simulink model "speedgoat_tcp_io"  (R2023a)
settings: Solver=FixedStepAuto  StartTime=0.0  StopTime=inf  RelTol=1e-3
model workspace (MAT data in the model file):
  outputs = {'uint8', 'uint8', 'uint8', 'uint8', 'uint8', 'uint8', 'uint8', 'uint8', 'double', 'double', 'double', 'double'}
undefined symbols (not defined in the file): Ended, Single
libraries: speedgoatlib_IO191 x5, slrealtimeiplib x3, slrealtimeutilitieslib x1, etargetslib x1
settings Model: Creator=tyler  LastModifiedBy=ivanl
settings SolverCC: ConcurrentTasks=on  PositivePriorityOrder=on
settings OptimizationCC: BlockReduction=off  OptimizeBlockIOStorage=off
settings DebuggingCC: TasksWithSamePriorityMsg=none
settings HardwareCC: ProdBitPerLong=64  ProdLongLongMode=on  ProdHWDeviceType=Intel->x86-64 (Linux 64)
settings RTWCC: Description=Simulink Real-Time  SystemTargetFile=slrealtime.tlc  TemplateMakefile=slrealtime_default_tmf  Toolchain=Simulink Real-Time Toolchain  BuildConfiguration=Faster Runs  CodeExecutionProfiling=on  TargetLang=C++

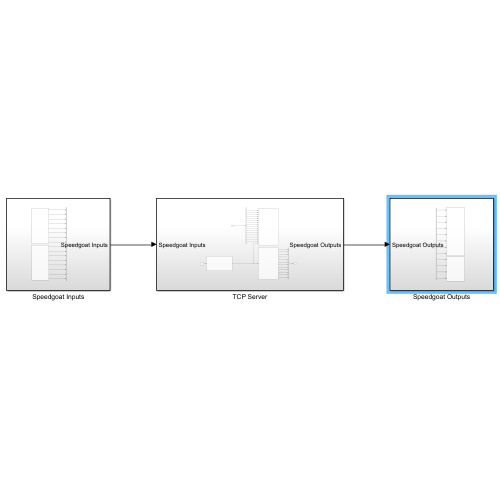
[thumbnail: Simulink's stored preview of the top-level diagram]
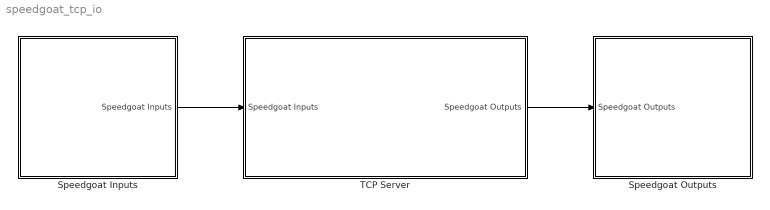
== system speedgoat_tcp_io ==
  Speedgoat Inputs : Subsystem
  Speedgoat Outputs : Subsystem
  TCP Server : Subsystem
  wires:
  Speedgoat Inputs/1(Speedgoat Inputs) -> TCP Server/1(Speedgoat Inputs)
  TCP Server/1(Speedgoat Outputs) -> Speedgoat Outputs/1(Speedgoat Outputs)

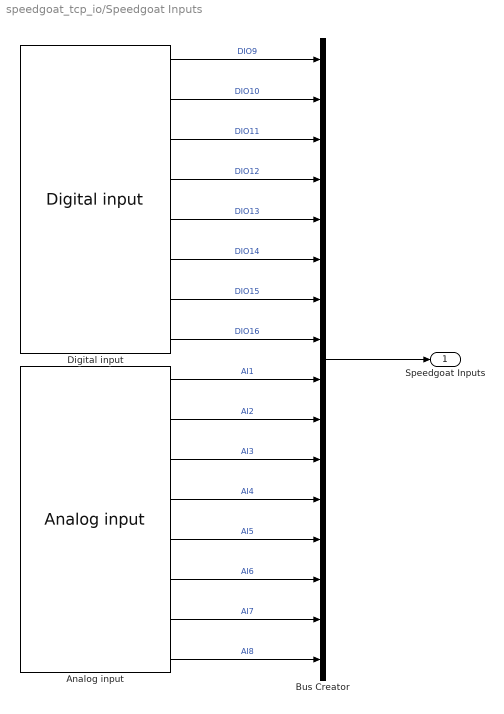
== system speedgoat_tcp_io/Speedgoat Inputs ==
  "Analog input " : speedgoatlib_IO191/Analog input   parModuleId=1  parSampleTime=-1  parPciSlot=-1  parAdcChannels=[1 2 3 4 5 6 7 8]  parAdcMode=2  parAdcRanges=[4 4 4 4 4 4 4 4]  parAdcInitValues=[0 0]  parAdcResets=[1 1]  paramsAdcDma=[0 1 200 -1]
      settings: SourceProductName=Simulink Real-Time: Speedgoat I/O Blockset
  Bus Creator : BusCreator  Inputs=16
  "Digital input " : speedgoatlib_IO191/Digital input   parModuleId=1  parSampleTime=-1  parPciSlot=-1  parDiChannels=[9 10 11 12 13 14 15 16]
      settings: SourceProductName=Simulink Real-Time: Speedgoat I/O Blockset
  Speedgoat Inputs : Outport
  wires:
  Bus Creator/1 -> Speedgoat Inputs/1
  "Digital input "/1 -> Bus Creator/1  "DIO9"
  "Digital input "/2 -> Bus Creator/2  "DIO10"
  "Digital input "/3 -> Bus Creator/3  "DIO11"
  "Digital input "/4 -> Bus Creator/4  "DIO12"
  "Digital input "/5 -> Bus Creator/5  "DIO13"
  "Digital input "/6 -> Bus Creator/6  "DIO14"
  "Digital input "/7 -> Bus Creator/7  "DIO15"
  "Digital input "/8 -> Bus Creator/8  "DIO16"
  "Analog input "/1 -> Bus Creator/9  "AI1"
  "Analog input "/2 -> Bus Creator/10  "AI2"
  "Analog input "/3 -> Bus Creator/11  "AI3"
  "Analog input "/4 -> Bus Creator/12  "AI4"
  "Analog input "/5 -> Bus Creator/13  "AI5"
  "Analog input "/6 -> Bus Creator/14  "AI6"
  "Analog input "/7 -> Bus Creator/15  "AI7"
  "Analog input "/8 -> Bus Creator/16  "AI8"

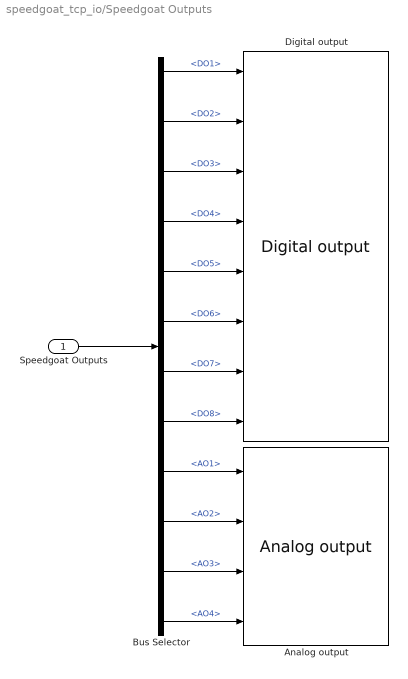
== system speedgoat_tcp_io/Speedgoat Outputs ==
  Speedgoat Outputs : Inport
  "Analog output " : speedgoatlib_IO191/Analog output   parModuleId=1  parSampleTime=-1  parPciSlot=-1  parDacChannels=[1 2 3 4]  parModuleType=1  parDacRanges=[3 3 3 3]  parDacInitValues=[0 0 0 0]  parDacResets=[1 1 1 1]
      settings: SourceProductName=Simulink Real-Time: Speedgoat I/O Blockset
  Bus Selector : BusSelector  OutputSignals=DO1,DO2,DO3,DO4,DO5,DO6,DO7,DO8,AO1,AO2,AO3,AO4
  "Digital output " : speedgoatlib_IO191/Digital output   parModuleId=1  parSampleTime=-1  parPciSlot=-1  parDoChannels=[1 2 3 4 5 6 7 8]  parDoInitValues=[0 0 0 0 0 0 0 0]  parDoResets=[1 1 1 1 1 1 1 1]
      settings: SourceProductName=Simulink Real-Time: Speedgoat I/O Blockset
  wires:
  Speedgoat Outputs/1 -> Bus Selector/1
  Bus Selector/4 -> "Digital output "/4  "<DO4>"
  Bus Selector/1 -> "Digital output "/1  "<DO1>"
  Bus Selector/2 -> "Digital output "/2  "<DO2>"
  Bus Selector/5 -> "Digital output "/5  "<DO5>"
  Bus Selector/3 -> "Digital output "/3  "<DO3>"
  Bus Selector/6 -> "Digital output "/6  "<DO6>"
  Bus Selector/7 -> "Digital output "/7  "<DO7>"
  Bus Selector/8 -> "Digital output "/8  "<DO8>"
  Bus Selector/9 -> "Analog output "/1  "<AO1>"
  Bus Selector/10 -> "Analog output "/2  "<AO2>"
  Bus Selector/11 -> "Analog output "/3  "<AO3>"
  Bus Selector/12 -> "Analog output "/4  "<AO4>"

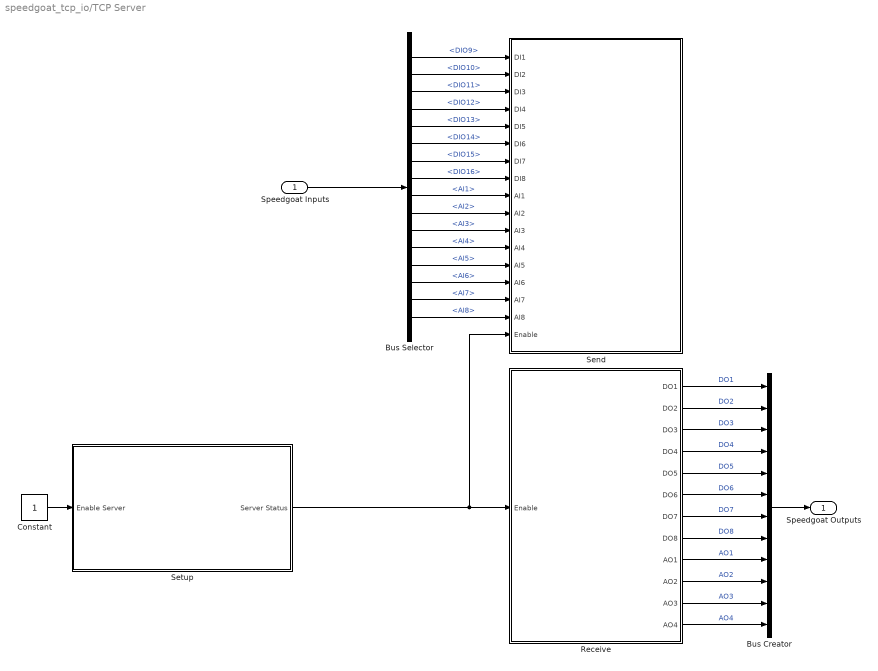
== system speedgoat_tcp_io/TCP Server ==
  Speedgoat Inputs : Inport
  Bus Creator : BusCreator  Inputs=12
  Bus Selector : BusSelector  OutputSignals=DIO9,DIO10,DIO11,DIO12,DIO13,DIO14,DIO15,DIO16,AI1,AI2,AI3,AI4,AI5,AI6,AI7,AI8
  Constant : Constant
  Receive : Subsystem
  Send : Subsystem
  Setup : Subsystem
  Speedgoat Outputs : Outport
  wires:
  Constant/1 -> Setup/1(Enable Server)
  Setup/1(Server Status) -> Send/17(Enable), Receive/1(Enable)
  Receive/1(DO1) -> Bus Creator/1  "DO1"
  Receive/2(DO2) -> Bus Creator/2  "DO2"
  Receive/3(DO3) -> Bus Creator/3  "DO3"
  Receive/4(DO4) -> Bus Creator/4  "DO4"
  Receive/5(DO5) -> Bus Creator/5  "DO5"
  Receive/6(DO6) -> Bus Creator/6  "DO6"
  Receive/7(DO7) -> Bus Creator/7  "DO7"
  Receive/8(DO8) -> Bus Creator/8  "DO8"
  Receive/9(AO1) -> Bus Creator/9  "AO1"
  Receive/10(AO2) -> Bus Creator/10  "AO2"
  Receive/11(AO3) -> Bus Creator/11  "AO3"
  Receive/12(AO4) -> Bus Creator/12  "AO4"
  Bus Creator/1 -> Speedgoat Outputs/1
  Speedgoat Inputs/1 -> Bus Selector/1
  Bus Selector/1 -> Send/1(DI1)  "<DIO9>"
  Bus Selector/2 -> Send/2(DI2)  "<DIO10>"
  Bus Selector/3 -> Send/3(DI3)  "<DIO11>"
  Bus Selector/4 -> Send/4(DI4)  "<DIO12>"
  Bus Selector/5 -> Send/5(DI5)  "<DIO13>"
  Bus Selector/6 -> Send/6(DI6)  "<DIO14>"
  Bus Selector/7 -> Send/7(DI7)  "<DIO15>"
  Bus Selector/8 -> Send/8(DI8)  "<DIO16>"
  Bus Selector/9 -> Send/9(AI1)  "<AI1>"
  Bus Selector/10 -> Send/10(AI2)  "<AI2>"
  Bus Selector/11 -> Send/11(AI3)  "<AI3>"
  Bus Selector/12 -> Send/12(AI4)  "<AI4>"
  Bus Selector/13 -> Send/13(AI5)  "<AI5>"
  Bus Selector/14 -> Send/14(AI6)  "<AI6>"
  Bus Selector/15 -> Send/15(AI7)  "<AI7>"
  Bus Selector/16 -> Send/16(AI8)  "<AI8>"

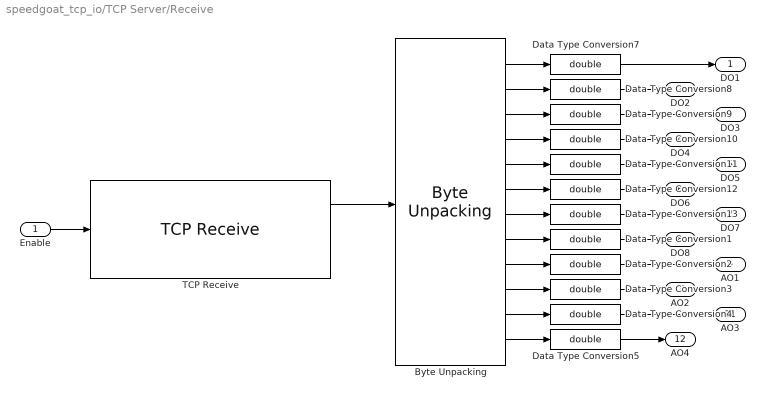
== system speedgoat_tcp_io/TCP Server/Receive ==
  Enable : Inport
  Byte Unpacking : slrealtimeutilitieslib/Byte Unpacking  MaskUnpackedDataTypes={'uint8','uint8','uint8','uint8','uint8','uint8','uint8','uint8','double','double','double','double'}  MaskUnpackedDataSizes={1,1,1,1,1,1,1,1,1,1,1,1}  MaskAlignment=1
  Data Type Conversion{1..5,7..13} (12 alike) : DataTypeConversion  OutDataTypeStr=double  SaturateOnIntegerOverflow=off  RndMeth=Floor
  TCP Receive : slrealtimeiplib/TCP Receive  socketAddPortVal=Server: 192.168.7.5:8001  rcvWidth=40  sampleTime=0.01
  DO1 : Outport
  DO2 : Outport  Port=2
  DO3 : Outport  Port=3
  DO4 : Outport  Port=4
  DO5 : Outport  Port=5
  DO6 : Outport  Port=6
  DO7 : Outport  Port=7
  DO8 : Outport  Port=8
  AO1 : Outport  Port=9
  AO2 : Outport  Port=10
  AO3 : Outport  Port=11
  AO4 : Outport  Port=12
  wires:
  Enable/1 -> TCP Receive/1
  TCP Receive/1 -> Byte Unpacking/1
  Byte Unpacking/8 -> Data Type Conversion1/1
  Byte Unpacking/7 -> Data Type Conversion13/1
  Byte Unpacking/2 -> Data Type Conversion8/1
  Byte Unpacking/6 -> Data Type Conversion12/1
  Data Type Conversion8/1 -> DO2/1
  Data Type Conversion10/1 -> DO4/1
  Data Type Conversion9/1 -> DO3/1
  Byte Unpacking/5 -> Data Type Conversion11/1
  Byte Unpacking/1 -> Data Type Conversion7/1
  Byte Unpacking/3 -> Data Type Conversion9/1
  Data Type Conversion12/1 -> DO6/1
  Byte Unpacking/10 -> Data Type Conversion3/1
  Byte Unpacking/9 -> Data Type Conversion2/1
  Byte Unpacking/4 -> Data Type Conversion10/1
  Data Type Conversion13/1 -> DO7/1
  Data Type Conversion11/1 -> DO5/1
  Byte Unpacking/12 -> Data Type Conversion5/1
  Data Type Conversion7/1 -> DO1/1
  Byte Unpacking/11 -> Data Type Conversion4/1
  Data Type Conversion1/1 -> DO8/1
  Data Type Conversion2/1 -> AO1/1
  Data Type Conversion3/1 -> AO2/1
  Data Type Conversion4/1 -> AO3/1
  Data Type Conversion5/1 -> AO4/1

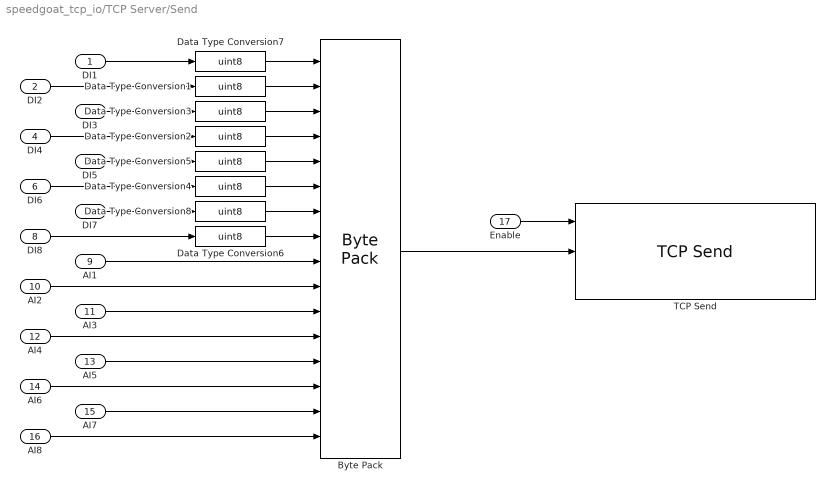
== system speedgoat_tcp_io/TCP Server/Send ==
  DI1 : Inport
  DI2 : Inport  Port=2
  DI3 : Inport  Port=3
  DI4 : Inport  Port=4
  DI5 : Inport  Port=5
  DI6 : Inport  Port=6
  DI7 : Inport  Port=7
  DI8 : Inport  Port=8
  AI1 : Inport  Port=9
  AI2 : Inport  Port=10
  AI3 : Inport  Port=11
  AI4 : Inport  Port=12
  AI5 : Inport  Port=13
  AI6 : Inport  Port=14
  AI7 : Inport  Port=15
  AI8 : Inport  Port=16
  Enable : Inport  Port=17
  Byte Pack : etargetslib/Byte Pack  datatypes={'uint8','uint8','uint8','uint8','uint8','uint8','uint8','uint8','double','double','double','double','double','double','double','double'}  byteAlign=1
  Data Type Conversion{1..8} (8 alike) : DataTypeConversion  OutDataTypeStr=uint8  SaturateOnIntegerOverflow=off  RndMeth=Floor
  TCP Send : slrealtimeiplib/TCP Send  socketAddPortVal=Server: 192.168.7.5:8001  sampleTime=0.01
  wires:
  Enable/1 -> TCP Send/1
  DI1/1 -> Data Type Conversion7/1
  DI2/1 -> Data Type Conversion1/1
  DI3/1 -> Data Type Conversion3/1
  DI4/1 -> Data Type Conversion2/1
  DI5/1 -> Data Type Conversion5/1
  DI6/1 -> Data Type Conversion4/1
  DI7/1 -> Data Type Conversion8/1
  DI8/1 -> Data Type Conversion6/1
  AI1/1 -> Byte Pack/9
  AI2/1 -> Byte Pack/10
  AI3/1 -> Byte Pack/11
  AI4/1 -> Byte Pack/12
  Byte Pack/1 -> TCP Send/2
  Data Type Conversion7/1 -> Byte Pack/1
  Data Type Conversion1/1 -> Byte Pack/2
  Data Type Conversion3/1 -> Byte Pack/3
  Data Type Conversion2/1 -> Byte Pack/4
  Data Type Conversion4/1 -> Byte Pack/6
  Data Type Conversion5/1 -> Byte Pack/5
  Data Type Conversion6/1 -> Byte Pack/8
  Data Type Conversion8/1 -> Byte Pack/7
  AI5/1 -> Byte Pack/13
  AI6/1 -> Byte Pack/14
  AI7/1 -> Byte Pack/15
  AI8/1 -> Byte Pack/16

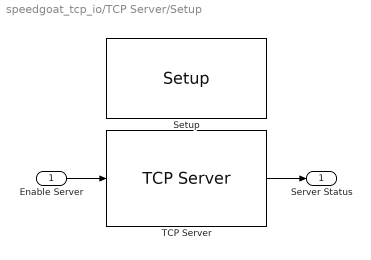
== system speedgoat_tcp_io/TCP Server/Setup ==
  Enable Server : Inport
  "Setup " : speedgoatlib_IO191/Setup   parModuleId=1  parPciSlot=-1  parTriggerSignal=TTL  parAdcChannels=[1 2 3 4 5 6 7 8]  parAdcRanges=[4 4 4 4 4 4 4 4]  parAdcChannel1=on  parAdcChannel2=on  parAdcChannel3=on  parAdcChannel4=on  parAdcChannel5=on  parAdcChannel6=on  parAdcChannel7=on  parAdcChannel8=on  parAdcMode=Single-Ended  parAdcRange11=+-5.12 V  parAdcRange21=+-24.576 V  parAdcRange12=+-5.12 V  parAdcRange22=+-24.576 V  parAdcRange13=+-5.12 V  parAdcRange23=+-24.576 V  parAdcRange14=+-5.12 V  parAdcRange24=+-24.576 V  parAdcRange15=+-5.12 V  parAdcRange25=+-24.576 V  parAdcRange16=+-5.12 V  parAdcRange26=+-24.576 V  parAdcRange17=+-5.12 V  parAdcRange27=+-24.576 V  parAdcRange18=+-5.12 V  parAdcRange28=+-24.576 V  parAdcEnDma=off  parAdcFrame=125  parAdcDiv=200  parAdcSample=-1  parDacChannels=[1 2 3 4]  parDacChannel1=on  parDacChannel2=on  parDacChannel3=on  parDacChannel4=on  parDacMode=Single-Ended  parDacRanges=[3 3 3 3]  parDacInitValues=[0 0 0 0]  parDacResets=[1 1 1 1]  parDacRange1=+-5 V  parDacInitValue1=0  parDacReset1=on  parDacRange2=+-5 V  parDacInitValue2=0  parDacReset2=on  parDacRange3=+-5 V  parDacInitValue3=0  parDacReset3=on  parDacRange4=+-5 V  parDacInitValue4=0  parDacReset4=on  parDiChannels=[9 10 11 12 13 14 15 16]  parDoChannels=[1 2 3 4 5 6 7 8]  parDioFirstControl=1  parDioSecondControl=0  parDioChannel1=Out  parExtra1=I  parExtra2=I  parExtra3=I  parDioChannel2=In  parDioChannel3=In  parDioChannel4=In  parDioChannel5=In  parDioChannel6=In  parDioChannel7=In  parDioChannel8=In  parDioChannel9=In  parDoInitValues=[0 0 0 0]  parDoResets=[1 1 1 1]  parDoInitValue1=0  parDoReset1=on  parDoInitValue2=0  parDoReset2=on  parDoInitValue3=0  parDoReset3=on  parDoInitValue4=0  parDoReset4=on  parDoInitValue5=0  parDoReset5=on  parDoInitValue6=0  parDoReset6=on  parDoInitValue7=0  parDoReset7=on  parDoInitValue8=0  parDoReset8=on  parDoInitValue9=0  parDoReset9=on  parDoInitValue10=0  parDoReset10=on  parDoInitValue11=0  parDoReset11=on  parDoInitValue12=0  parDoReset12=on  parDoInitValue13=0  parDoReset13=on  parDoInitValue14=0  parDoReset14=on  parDoInitValue15=0  parDoReset15=on  parDoInitValue16=0  parDoReset16=on
      settings: SourceProductName=Simulink Real-Time: Speedgoat I/O Blockset
  TCP Server : slrealtimeiplib/TCP Server  Priority=-1  useHostTargetConn=off  serverAddress=192.168.7.5  serverPort=8001
  Server Status : Outport
  wires:
  Enable Server/1 -> TCP Server/1
  TCP Server/1 -> Server Status/1
